simulink model "nauni_fieldtesting"  (R2025b)
settings: Solver=FixedStepDiscrete  StartTime=0.0  StopTime=86400  FixedStep=1  RelTol=1e-3
InitFcn:
  | init_nauni;
  | set_param(bdroot,'StopTime',num2str(StopTime));
undefined symbols (not defined in the file): a, a_soil, DiscIntNeverNeededParam, evap_rate, noise, rain_every_hours, rain_pulse, RH_amp, RH_mean, T_amp, T_mean, Ts, Tsoil_amp, Tsoil_lag_h, Tsoil_mean, VWC_init, VWC_max, VWC_min
libraries: simulink x4
settings Model: Creator=Hunny  LastModifiedBy=Hunny
settings DataIOCC: SaveState=on

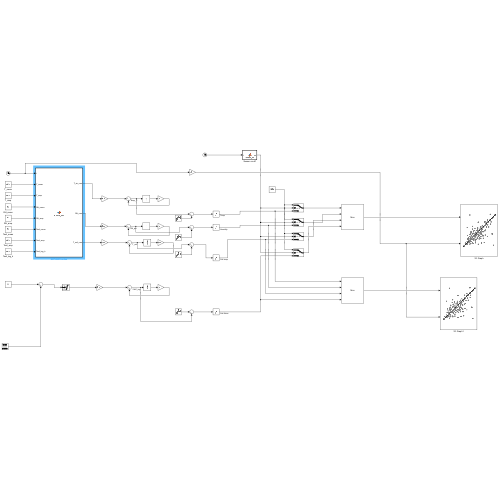
[thumbnail: Simulink's stored preview of the top-level diagram]
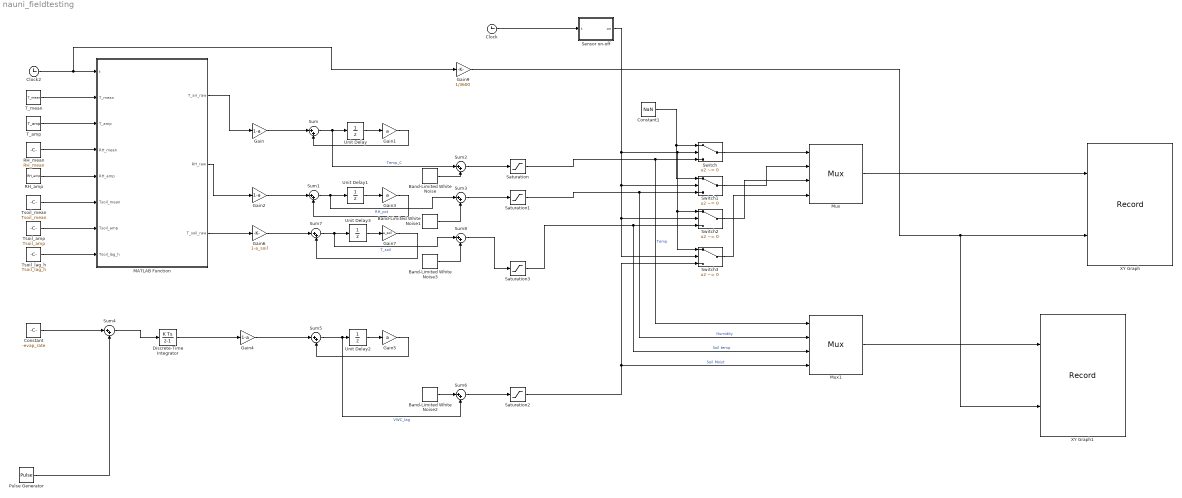
== system nauni_fieldtesting ==
  Band-Limited White Noise : simulink/Sources/Band-Limited White Noise  Cov=noise.T^2  Ts=Ts  seed=[23341]
  Band-Limited White Noise1 : simulink/Sources/Band-Limited White Noise  Cov=noise.RH^2  Ts=Ts  seed=[23341]
  Band-Limited White Noise2 : simulink/Sources/Band-Limited White Noise  Cov=noise.VWC^2,  Ts=Ts  seed=[23341]
  Band-Limited White Noise3 : simulink/Sources/Band-Limited White Noise  Cov=noise.Tsoil^2  Ts=Ts  seed=[23341]
  Clock : Clock
  Clock2 : Clock
  Constant : Constant  Value=-evap_rate  SampleTime=Ts
  Constant1 : Constant  Value=NaN
  Discrete-Time Integrator : DiscreteIntegrator  InitialCondition=VWC_init  SampleTime=Ts  LimitOutput=on  ICPrevOutput=DiscIntNeverNeededParam  ICPrevScaledInput=DiscIntNeverNeededParam
  Gain : Gain  Gain=1-a
  Gain1 : Gain  Gain=a
  Gain2 : Gain  Gain=1-a
  Gain3 : Gain  Gain=a
  Gain4 : Gain  Gain=1-a
  Gain5 : Gain  Gain=a
  Gain6 : Gain  Gain=1-a_soil
  Gain7 : Gain  Gain=a_soil
  Gain9 : Gain  Gain=1/3600
  MATLAB Function : MATLAB Function  TreatAsAtomicUnit=on
  Mux : Mux
  Mux1 : Mux
  Pulse Generator : DiscretePulseGenerator  Amplitude=rain_pulse  Period=rain_every_hours*1800  SampleTime=Ts
  RH_amp : Constant  Value=RH_amp
  RH_mean : Constant  Value=RH_mean
  Saturation : Saturate  UpperLimit=50  LowerLimit=-10
  Saturation1 : Saturate  UpperLimit=100  LowerLimit=30
  Saturation2 : Saturate  UpperLimit=VWC_max  LowerLimit=VWC_min
  Saturation3 : Saturate  UpperLimit=40  LowerLimit=0
  Sensor on-off : MATLAB Function  TreatAsAtomicUnit=on
  Sum{,1..8} (9 alike) : Sum  Inputs=|++
  Switch{,1..3} (4 alike) : Switch  Criteria=u2 ~= 0  SaturateOnIntegerOverflow=off  InputSameDT=off
  T_amp : Constant  Value=T_amp
  T_mean : Constant  Value=T_mean
  Tsoil_amp : Constant  Value=Tsoil_amp
  Tsoil_lag_h : Constant  Value=Tsoil_lag_h
  Tsoil_mean : Constant  Value=Tsoil_mean
  Unit Delay{,1..3} (4 alike) : UnitDelay  SampleTime=Ts  HasFrameUpgradeWarning=on
  XY Graph : Record  NumPorts=2.0  RecordToWorkspace=on  FileSettingsInternal="{\"entries\":[{\"content\":{\"excelSettings\":{\"content\":{},\"type\":\"Streamout.ExcelSettings\"},\"parquetSettings\":{\"content\":{},\"type\":\"Streamout.ParquetSettings\"}},\"type\":\"Streamout.FileSettingStorage\",\"uuid\":\"\"}],\"packageUris\":[\"http:\\/\\/schema.mathworks.com\\/mf0\\/streamout_blocks\\/R2020a\"],\"version\":\"1.0\"}"  FrameSettings=[0, 0]  Layout=[1 1]  SignalsInternal="{\"entries\":[{\"content\":{},\"type\":\"RecordBlkView.InputSignals\",\"uuid\":\"\"}],\"packageUris\":[\"http:\\/\\/schema.mathworks.com\\/mf0\\/streamout_blocks\\/R2020a\"],\"version\":\"1.0\"}"  VisualizationBindings="{\"xyplotplugin\":{\"info\":[{\"series\":[{\"bindingParametersList\":[{\"parameter\":\"X-Axis\",\"signalID\":277,\"signalName\":\"Gain9\"},{\"parameter\":\"Y-Axis\",\"signalID\":273,\"signalName\":\"Mux(1)\"}],\"seriesID\":0},{\"bindingParametersList\":[{\"parameter\":\"X-Axis\",\"signalID\":277,\"signalName\":\"Gain9\"},{\"parameter\":\"Y-Axis\",\"signalID\":311,\"signalName\":\"Mux(2)\"}],\"seriesID\":1},{\"bindingParametersList\":[{\"parameter\":\"X-Axis\",\"signalID\":277,\"signalName\":\"Gain9\"},{\"parameter\":\"Y-Axis\",\"signalID\":312,\"signalName\":\"Mux(3)\"}],\"seriesID\":2},{\"bindingParametersList\":[{\"parameter\":\"X-Axis\",\"signalID\":277,\"signalName\":\"Gain9\"},{\"parameter\":\"Y-Axis\",\"signalID\":313,\"signalName\":\"Mux(4)\"}],\"seriesID\":3}],\"subplotID\":1}]}}"  CompatibilityTag=XY
  XY Graph1 : Record  NumPorts=2.0  FileSettingsInternal="{\"entries\":[{\"content\":{\"excelSettings\":{\"content\":{},\"type\":\"Streamout.ExcelSettings\"},\"parquetSettings\":{\"content\":{},\"type\":\"Streamout.ParquetSettings\"}},\"type\":\"Streamout.FileSettingStorage\",\"uuid\":\"\"}],\"packageUris\":[\"http:\\/\\/schema.mathworks.com\\/mf0\\/streamout_blocks\\/R2020a\"],\"version\":\"1.0\"}"  FrameSettings=[0, 0]  Layout=[1 1]  SignalsInternal="{\"entries\":[{\"content\":{\"signals\":[{\"content\":{\"blockPath\":[],\"dimensions\":[4],\"domain\":\"\",\"hasChildren\":true,\"lineColor\":\"#d95319\",\"lineWidth\":2,\"port\":1,\"sid\":[\"\"],\"signalID\":1,\"signalName\":\"Mux\"},\"type\":\"RecordBlkView.Signal\",\"uuid\":\"\"},{\"content\":{\"blockPath\":[],\"channel\":[1],\"dimensions\":[4],\"domain\":\"\",\"lineColor\":\"#7e2f8e\",\"lineWidth\":2,\"parentID\":1,\"port\":1,\"sid\":[\"\"],\"signalID\":2,\"signalName\":\"Mux\"},\"type\":\"RecordBlkView.Signal\",\"uuid\":\"\"},{\"content\":{\"blockPath\":[],\"dimensions\":[1],\"domain\":\"\",\"lineColor\":\"#ffffff\",\"port\":2,\"sid\":[\"\"],\"signalID\":3,\"signalName\":\"Gain9\"},\"type\":\"RecordBlkView.Signal\",\"uuid\":\"\"},{\"content\":{\"blockPath\":[],\"dimensions\":[4],\"domain\":\"\",\"hasChildren\":true,\"lineColor\":\"#77ac30\",\"lineWidth\":2,\"port\":1,\"sid\":[\"\"],\"signalID\":4,\"signalName\":\"Mux1\"},\"type\":\"RecordBlkView.Signal\",\"uuid\":\"\"},{\"content\":{\"blockPath\":[],\"channel\":[1],\"dimensions\":[4],\"domain\":\"\",\"lineColor\":\"#7e2f8e\",\"lineWidth\":2,\"parentID\":4,\"plots\":[ 1 ],\"port\":1,\"sid\":[\"\"],\"signalID\":5,\"signalName\":\"Mux1\"},\"type\":\"RecordBlkView.Signal\",\"uuid\":\"\"},{\"content\":{\"blockPath\":[],\"dimensions\":[1],\"domain\":\"\",\"lineColor\":\"#ffffff\",\"plots\":[ 1 ],\"port\":2,\"sid\":[\"\"],\"signalID\":6,\"signalName\":\"Gain9\"},\"type\":\"RecordBlkView.Signal\",\"uuid\":\"\"},{\"content\":{\"blockPath\":[],\"dimensions\":[1],\"domain\":\"\",\"lineColor\":\"#77ac30\",\"lineWidth\":2,\"sid\":[\"\"],\"signalID\":7,\"signalName\":\"DSTATE\"},\"type\":\"RecordBlkView.Signal\",\"uuid\":\"\"},{\"content\":{\"blockPath\":[],\"dimensions\":[1],\"domain\":\"\",\"lineColor\":\"#4dbeee\",\"lineWidth\":2,\"sid\":[\"\"],\"signalID\":8,\"signalName\":\"DSTATE\"},\"type\":\"RecordBlkView.Signal\",\"uuid\":\"\"},{\"content\":{\"blockPath\":[],\"dimensions\":[1],\"domain\":\"\",\"lineColor\":\"#a2142f\",\"lineWidth\":2,\"sid\":[\"\"],\"signalID\":9,\"signalName\":\"DSTATE\"},\"type\":\"RecordBlkView.Signal\",\"uuid\":\"\"},{\"content\":{\"blockPath\":[],\"dimensions\":[1],\"domain\":\"\",\"lineColor\":\"#139fff\",\"lineWidth\":2,\"sid\":[\"\"],\"signalID\":10,\"signalName\":\"DSTATE\"},\"type\":\"RecordBlkView.Signal\",\"uuid\":\"\"},{\"content\":{\"blockPath\":[],\"dimensions\":[1],\"domain\":\"\",\"lineColor\":\"#ff6929\",\"lineWidth\":2,\"sid\":[\"\"],\"signalID\":11,\"signalName\":\"DSTATE\"},\"type\":\"RecordBlkView.Signal\",\"uuid\":\"\"},{\"content\":{\"blockPath\":[],\"channel\":[2],\"dimensions\":[4],\"domain\":\"\",\"lineColor\":\"#64d413\",\"lineWidth\":2,\"parentID\":1,\"port\":1,\"sid\":[\"\"],\"signalID\":12,\"signalName\":\"Mux\"},\"type\":\"RecordBlkView.Signal\",\"uuid\":\"\"},{\"content\":{\"blockPath\":[],\"channel\":[3],\"dimensions\":[4],\"domain\":\"\",\"lineColor\":\"#a2142f\",\"lineWidth\":2,\"parentID\":1,\"port\":1,\"sid\":[\"\"],\"signalID\":13,\"signalName\":\"Mux\"},\"type\":\"RecordBlkView.Signal\",\"uuid\":\"\"},{\"content\":{\"blockPath\":[],\"channel\":[4],\"dimensions\":[4],\"domain\":\"\",\"lineColor\":\"#fe330a\",\"lineWidth\":2,\"parentID\":1,\"port\":1,\"sid\":[\"\"],\"signalID\":14,\"signalName\":\"Mux\"},\"type\":\"RecordBlkView.Signal\",\"uuid\":\"\"},{\"content\":{\"blockPath\":[],\"channel\":[2],\"dimensions\":[4],\"domain\":\"\",\"lineColor\":\"#64d413\",\"lineWidth\":2,\"parentID\":4,\"plots\":[ 1 ],\"port\":1,\"sid\":[\"\"],\"signalID\":15,\"signalName\":\"Mux1\"},\"type\":\"RecordBlkView.Signal\",\"uuid\":\"\"},{\"content\":{\"blockPath\":[],\"channel\":[3],\"dimensions\":[4],\"domain\":\"\",\"lineColor\":\"#a2142f\",\"lineWidth\":2,\"parentID\":4,\"plots\":[ 1 ],\"port\":1,\"sid\":[\"\"],\"signalID\":16,\"signalName\":\"Mux1\"},\"type\":\"RecordBlkView.Signal\",\"uuid\":\"\"},{\"content\":{\"blockPath\":[],\"channel\":[4],\"dimensions\":[4],\"domain\":\"\",\"lineColor\":\"#fe330a\",\"lineWidth\":2,\"parentID\":4,\"plots\":[ 1 ],\"port\":1,\"sid\":[\"\"],\"signalID\":17,\"signalName\":\"Mux1\"},\"type\":\"RecordBlkView.Signal\",\"uuid\":\"\"}]},\"type\":\"RecordBlkView.InputSignals\",\"uuid\":\"\"}],\"packageUris\":[\"http:\\/\\/schema.mathworks.com\\/mf0\\/streamout_blocks\\/R2020a\"],\"version\":\"1.0\"}"  VisualizationBindings="{\"xyplotplugin\":{\"info\":[{\"series\":[{\"bindingParametersList\":[{\"parameter\":\"X-Axis\",\"signalID\":6,\"signalName\":\"Gain9\"},{\"parameter\":\"Y-Axis\",\"signalID\":5,\"signalName\":\"Mux1(1)\"}],\"seriesID\":0},{\"bindingParametersList\":[{\"parameter\":\"X-Axis\",\"signalID\":6,\"signalName\":\"Gain9\"},{\"parameter\":\"Y-Axis\",\"signalID\":15,\"signalName\":\"Mux1(2)\"}],\"seriesID\":1},{\"bindingParametersList\":[{\"parameter\":\"X-Axis\",\"signalID\":6,\"signalName\":\"Gain9\"},{\"parameter\":\"Y-Axis\",\"signalID\":16,\"signalName\":\"Mux1(3)\"}],\"seriesID\":2},{\"bindingParametersList\":[{\"parameter\":\"X-Axis\",\"signalID\":6,\"signalName\":\"Gain9\"},{\"parameter\":\"Y-Axis\",\"signalID\":17,\"signalName\":\"Mux1(4)\"}],\"seriesID\":3}],\"subplotID\":1}]}}"  CompatibilityTag=XY
  wires:
  T_mean/1 -> MATLAB Function/2(T_mean)
  T_amp/1 -> MATLAB Function/3(T_amp)
  RH_mean/1 -> MATLAB Function/4(RH_mean)
  RH_amp/1 -> MATLAB Function/5(RH_amp)
  MATLAB Function/1(T_air_raw) -> Gain/1
  Gain/1 -> Sum/1
  Sum/1 -> Sum2/1, Unit Delay/1  "Temp_C"
  MATLAB Function/2(RH_raw) -> Gain2/1
  Gain2/1 -> Sum1/1
  Sum1/1 -> Sum3/1, Unit Delay1/1  "RH_pct"
  Unit Delay/1 -> Gain1/1
  Gain1/1 -> Sum/2
  Unit Delay1/1 -> Gain3/1
  Gain3/1 -> Sum1/2
  Band-Limited White Noise/1 -> Sum2/2
  Sum2/1 -> Saturation/1
  Band-Limited White Noise1/1 -> Sum3/2
  Sum3/1 -> Saturation1/1
  Constant/1 -> Sum4/1
  Pulse Generator/1 -> Sum4/2
  Sum4/1 -> Discrete-Time Integrator/1
  Sum5/1 -> Sum6/2, Unit Delay2/1  "VWC_lag"
  Unit Delay2/1 -> Gain5/1
  Gain5/1 -> Sum5/2
  Band-Limited White Noise2/1 -> Sum6/1
  Sum6/1 -> Saturation2/1
  Saturation/1 -> Mux1/1, Switch/3  "Temp"
  Mux/1 -> XY Graph/1
  Saturation1/1 -> Mux1/2, Switch1/3  "Humidity"
  Saturation2/1 -> Mux1/4, Switch3/3  "Soil Moist"
  Discrete-Time Integrator/1 -> Gain4/1
  Gain4/1 -> Sum5/1
  Tsoil_mean/1 -> MATLAB Function/6(Tsoil_mean)
  Tsoil_amp/1 -> MATLAB Function/7(Tsoil_amp)
  Tsoil_lag_h/1 -> MATLAB Function/8(Tsoil_lag_h)
  Gain6/1 -> Sum7/1
  Sum7/1 -> Sum8/1, Unit Delay3/1  "T_soil"
  Unit Delay3/1 -> Gain7/1
  Gain7/1 -> Sum7/2
  Band-Limited White Noise3/1 -> Sum8/2
  Sum8/1 -> Saturation3/1
  MATLAB Function/3(T_soil_raw) -> Gain6/1
  Saturation3/1 -> Mux1/3, Switch2/3  "Soil temp"
  Clock2/1 -> Gain9/1, MATLAB Function/1(t)
  Gain9/1 -> XY Graph1/2, XY Graph/2
  Clock/1 -> Sensor on-off/1(t)
  Sensor on-off/1(on) -> Switch3/2, Switch2/2, Switch1/2, Switch3/1, Switch2/1, Switch/2
  Constant1/1 -> Switch1/1, Switch/1
  Switch/1 -> Mux/1
  Switch1/1 -> Mux/2
  Switch2/1 -> Mux/3
  Switch3/1 -> Mux/4
  Mux1/1 -> XY Graph1/1

== matlab function nauni_fieldtesting/Sensor on-off ==
  data: t input; on output
function on = sensor_on(t)
% t is simulation time in seconds
period = 31*60;   % total cycle: 31 minutes = 60s on + 30min off
awake  = 60;      % 60 seconds active

phase = mod(t, period);   % position within each 31-min cycle
if phase < awake
    on = 0;    % sensor awake (1 min)
else
    on = 1;    % sensor sleeping (30 min)
end
end

== matlab function nauni_fieldtesting/MATLAB Function ==
  data: t input; T_air_raw output; T_mean input; T_amp input; RH_mean input; RH_amp input; RH_raw output; Tsoil_mean input; Tsoil_amp input; Tsoil_lag_h input; T_soil_raw output
function [T_air_raw, RH_raw, T_soil_raw] = diurnal_env( ...
    t, T_mean, T_amp, RH_mean, RH_amp, ...
    Tsoil_mean, Tsoil_amp, Tsoil_lag_h)

hr = mod(t/3600, 24);

% Air temperature
T_air_raw = T_mean + T_amp * sin(2*pi*(hr - 5)/24);

% Relative humidity
RH_raw = RH_mean + RH_amp * sin(2*pi*(hr + 7)/24);

% Soil temperature: delayed & smaller swing
T_soil_raw = Tsoil_mean + Tsoil_amp * ...
             sin(2*pi*(hr - 5 - Tsoil_lag_h)/24);
end
